simulink model "modulation01"  (R2015a)
settings: Solver=ode45  StartTime=0.0  StopTime=30  RelTol=1e-3
undefined symbols (not defined in the file): fdesignblkfcn, gcbh
libraries: dspsnks4 x1
settings Model: Creator=ekulasek  LastModifiedBy=chulantha

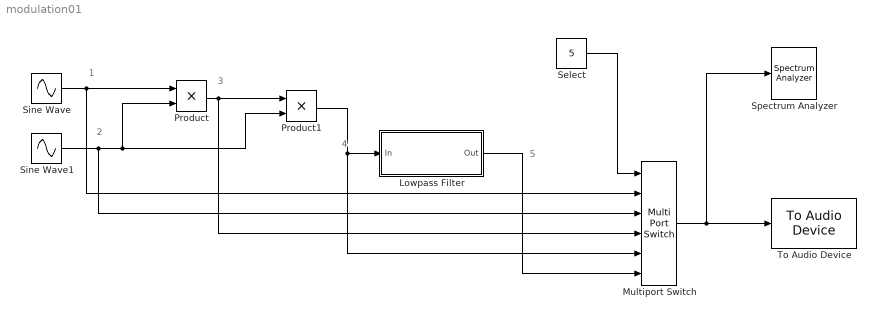
== system modulation01 ==
  note: 5
  note: 4
  note: 3
  note: 2
  note: 1
  Lowpass Filter : Subsystem  DialogController=fdesignblkfcn  InitFcn=fdesignblkfcn(gcbh, {'InitFcn'});  mask(Lowpass Filter){}
      mask help: Design a lowpass filter
      settings: CopyFcn=fdesignblkfcn(gcbh, {'CopyFcn'});
      mask Help: helpview(mapfilelocation('dsp'), 'dsplowpassfilter');
      mask Display: disp('Lowpass')
  Multiport Switch : MultiPortSwitch  Inputs=5
  Product : Product
  Product1 : Product
  Select : Constant  Value=5
  Sine Wave : Sin  SineType=Sample based  Frequency=2*pi*22  Samples=round(44100/500)  SampleTime=1/44100
  Sine Wave1 : Sin  SineType=Sample based  Frequency=2*pi*1000  Samples=round(44100/5000)  SampleTime=1/44100
  Spectrum Analyzer : SpectrumAnalyzer
  To Audio Device : dspsnks4/To Audio Device  deviceName=Default  inheritSampleRate=on  sampleRate=44100  deviceDatatype=Determine from input data type  autoBufferSize=on  bufferSize=4096  queueDuration=1.0  defaultOutputChannelMapping=on  outputChannelMapping=1:2  outputNumUnderrunSamples=off
  wires:
  Sine Wave1/1 -> Multiport Switch/3, Product/2, Product1/2
  Sine Wave/1 -> Multiport Switch/2, Product/1
  Product/1 -> Multiport Switch/4, Product1/1
  Product1/1 -> Multiport Switch/5, Lowpass Filter/1(In)
  Lowpass Filter/1(Out) -> Multiport Switch/6
  Multiport Switch/1 -> Spectrum Analyzer/1, To Audio Device/1
  Select/1 -> Multiport Switch/1

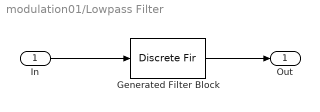
== system modulation01/Lowpass Filter ==
  In : Inport
  Generated Filter Block : DiscreteFir  Tag=BlockMethodSubSystem  Coefficients=[-1.18554501911034474e-07 -4.89279276613347799e-07 -1.44794172326237458e-06 -3.55818056274897542e-06 -7.72746958942818345e-06 -1.53153366595587155e-05 -2.82369124265530089e-05 -4.90398217198297355e-05 -8.09272654466181295e-05 -0.000127697735756357174 -0.000193571929466272578 -0.000282882607628189876 -0.000399615452997945011 -0.000546806022810973754 -0.000725821478047858001 -0.000935582868897918149 -0.00117181049314795511 -0.00142639900902543347 -0.00168704431944994649 -0.00193724629696120573 -0.00215679698846420968 -0.0023228296426153084 -0.00241144997593303965 -0.00239990041056007417 -0.00226912647199739928 -0.00200653100241507572 -0.00160862753337246843 -0.00108325206965011037 -0.000450974191819739599 0.000254626512982162646 0.000988077946539570214 0.0016946625900483563 0.0023145646317095773 0.00278829475470533314 0.0030629708325114937 0.00309885243109220233 0.00287539316033127643 0.00239601316952048771 0.00169082476075412317 0.000816678365507536824 -0.000145867514291889204 -0.00109872556629794739 -0.00193530049945775449 -0.00255164700358367262 -0.00285869702884691259 -0.00279421104274031997 -0.00233296433221999791 -0.00149370640963797309 -0.000341648310999295224 0.00101436443168914214 0.00243027469796616193 0.00374044880579517229 0.00477544306491543488 0.0053821788644584324 0.00544430455502436898 0.00490024786694244138 0.0037564727338225282 0.00209377953739782853 6.51206847552656461e-05 -0.00211570365457531238 -0.00419403791857668549 -0.00590149618735953153 -0.00698762004827387009 -0.00725264363026099229 -0.00657745753285743275 -0.00494681685982934459 -0.00246227453445260758 0.000657770736235516033 0.00409221222489680302 0.00744527292987279526 0.0102864664346131902 0.0121989052183728956 0.0128310755792072559 0.0119463671869925493 0.00946442372000739357 0.00548883999279767189 0.00031686386115062522 -0.00557152022475916262 -0.0115456089395913845 -0.016875244397574117 -0.0207971958770402469 -0.0225905856812901491 -0.0216539143501210743 -0.0175756281944941702 -0.0101904257572652049 0.000385370357933679554 0.0137441347694759429 0.0292051970296891769 0.0458604245243913952 0.0626436333104862103 0.0784177325771640427 0.0920714959079848155 0.1026166605003105 0.109275831551216215 0.111552453647841596 0.109275831551216215 0.1026166605003105 0.0920714959079848155 0.0784177325771640427 0.0626436333104862103 0.0458604245243913952 0.0292051970296891769 0.0137441347694759429 0.000385370357933679554 -0.0101904257572652049 -0.0175756281944941702 -0.0216539143501210743 -0.0225905856812901491 -0.0207971958770402469 -0.016875244397574117 -0.0115456089395913845 -0.00557152022475916262 0.00031686386115062522 0.00548883999279767189 0.00946442372000739357 0.0119463671869925493 0.0128310755792072559 0.0121989052183728956 0.0102864664346131902 0.00744527292987279526 0.00409221222489680302 0.000657770736235516033 -0.00246227453445260758 -0.00494681685982934459 -0.00657745753285743275 -0.00725264363026099229 -0.00698762004827387009 -0.00590149618735953153 -0.00419403791857668549 -0.00211570365457531238 6.51206847552656461e-05 0.00209377953739782853 0.0037564727338225282 0.00490024786694244138 0.00544430455502436898 0.0053821788644584324 0.00477544306491543488 0.00374044880579517229 0.00243027469796616193 0.00101436443168914214 -0.000341648310999295224 -0.00149370640963797309 -0.00233296433221999791 -0.00279421104274031997 -0.00285869702884691259 -0.00255164700358367262 -0.00193530049945775449 -0.00109872556629794739 -0.000145867514291889204 0.000816678365507536824 0.00169082476075412317 0.00239601316952048771 0.00287539316033127643 0.00309885243109220233 0.0030629708325114937 0.00278829475470533314 0.0023145646317095773 0.0016946625900483563 0.000988077946539570214 0.000254626512982162646 -0.000450974191819739599 -0.00108325206965011037 -0.00160862753337246843 -0.00200653100241507572 -0.00226912647199739928 -0.00239990041056007417 -0.00241144997593303965 -0.0023228296426153084 -0.00215679698846420968 -0.00193724629696120573 -0.00168704431944994649 ...(+448 chars)]  InputProcessing=Columns as channels (frame based)
  Out : Outport
  wires:
  In/1 -> Generated Filter Block/1
  Generated Filter Block/1 -> Out/1
